simulink model "sol2"  (R2021b)
settings: Solver=VariableStepAuto  StartTime=0.0  StopTime=1  RelTol=1e-3
PreLoadFcn:
  | initModelData
values from neighbouring files (symbols this model uses):
  B = Bm+(Kb*Km/R)    (= 0.0149065789474)    [MyData_for_1_and_2.m]    (also in MyData_for_3_4_and_5.m; MyData_for_5_and_6.m)
  Jm = 5.5e-4    (= 0.00055)    [MyData_for_1_and_2.m]    (also in MyData_for_3_4_and_5.m; MyData_for_5_and_6.m)
  Km = 0.105    [MyData_for_1_and_2.m]    (also in MyData_for_3_4_and_5.m; MyData_for_5_and_6.m)
  r = 156    [MyData_for_1_and_2.m]    (also in MyData_for_3_4_and_5.m; MyData_for_5_and_6.m)
  R = 0.76    [MyData_for_1_and_2.m]    (also in MyData_for_3_4_and_5.m; MyData_for_5_and_6.m)
settings Model: Creator=esdan  LastModifiedBy=munir
settings SolverCC: AlgebraicLoopSolver=TrustRegion
settings DebuggingCC: SFMachineParentedDataDiag=warning

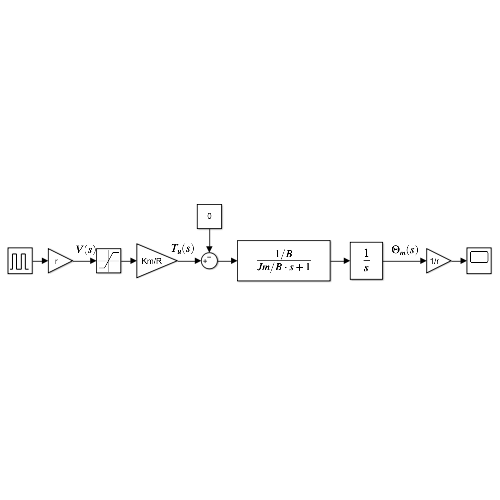
[thumbnail: Simulink's stored preview of the top-level diagram]
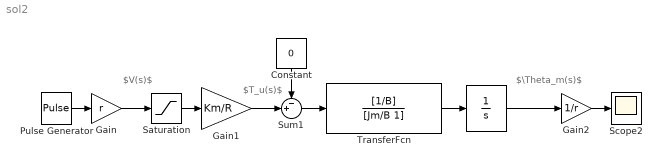
== system sol2 ==
  note: $\Theta_m(s)$
  note: $V(s)$
  note: $T_u(s)$
  " " : Integrator
  Constant : Constant  Value=0
  Gain : Gain  Gain=r
  Gain1 : Gain  Gain=Km/R
  Gain2 : Gain  Gain=1/r
  Pulse Generator : DiscretePulseGenerator  PulseType=Time based  Period=1  PulseWidth=50
  Saturation : Saturate  UpperLimit=35  LowerLimit=-35
  Scope2 : Scope
  Sum1 : Sum  Inputs=-+|
  TransferFcn : TransferFcn  Numerator=[1/B]  Denominator=[Jm/B 1]
  wires:
  TransferFcn/1 -> " "/1
  Saturation/1 -> Gain1/1
  Gain1/1 -> Sum1/2
  Sum1/1 -> TransferFcn/1
  Constant/1 -> Sum1/1
  Gain/1 -> Saturation/1
  " "/1 -> Gain2/1
  Gain2/1 -> Scope2/1
  Pulse Generator/1 -> Gain/1
